simulink model "Sim_v19_PL0001_checkSignConv"  (R2015a)
settings: Solver=ode4  StartTime=0.0  StopTime=300  FixedStep=Ts  RelTol=1e-3
PreLoadFcn:
  | Ts=0.1;
PostLoadFcn:
  | Ts=0.1;
InitFcn:
  | Ts=0.1;
StartFcn:
  | Ts=0.1;
values from neighbouring files (symbols this model uses):
  ctrl_idx = strToIdx(actStr,loadNames)    [Driver_PL0001.m]
  dbc_idx = strToIdx(dbcStr,loadNames)    [Driver_PL0001.m]
  Ki_vang = Ki_vang*5    [Driver_PL0001.m]    (also in afunc.m = zeros(r,1))
  Ki_vmag = Ki_vmag*5    [Driver_PL0001.m]    (also in afunc.m = zeros(r,1))
  Kp_vang = Kp_vang*5    [Driver_PL0001.m]    (also in afunc.m = zeros(r,1))
  Kp_vmag = Kp_vmag*5    [Driver_PL0001.m]    (also in afunc.m = zeros(r,1))
  meas_idx = strToIdx(measStr,busNames)    [Driver_PL0001.m]
  ridx = ridx(~isnan(ridx))    [Driver_PL0001.m]
  Sinv = repmat(Sinv_str,1,length(ctrl_idx)/2)    [Driver_PL0001.m]
  Vang_ctrlStart = (20+80*r)*Ts    [Driver_PL0001.m]
  vang_init_actual = vang_new(4,:)    [Driver_PL0001.m]    (also in PlotLocalCtrl_May15.m = [[0:60:(minEnd-minStart)*60]',repmat(vang_new(2,:),minEnd-mi; PlotLocalCtrl_May15_2ph.m = [[0:60:(minEnd-minStart)*60]',repmat(vang_new(2,:),minEnd-mi; set_const_target.m = Vang_nom)
  Vmag_ctrlStart = (20+80*r)*Ts    [Driver_PL0001.m]
  vmag_init_actual = vmag_new(4,:)    [Driver_PL0001.m]    (also in PlotLocalCtrl_May15.m = [[0:60:(minEnd-minStart)*60]',repmat(vmag_new(2,:),minEnd-mi; PlotLocalCtrl_May15_2ph.m = [[0:60:(minEnd-minStart)*60]',repmat(vmag_new(2,:),minEnd-mi; set_const_target.m = Vmag_nom)
undefined symbols (not defined in the file or in its folder): Sbase, V1base
libraries: dspindex x9, opal_lib x2, rtlab x2, rtlab_phasor x1
settings Model: Creator=Jaimie.Swartz  LastModifiedBy=Jaimie.Swartz
settings SolverCC: AlgebraicLoopSolver=LineSearch
settings DataIOCC: SignalLoggingSaveFormat=ModelDataLogs  SignalLogging=off  DSMLogging=off  VisualizeSimOutput=off
settings OptimizationCC: ExpressionDepthLimit=2147483647
settings DebuggingCC: UnderspecifiedInitializationDetection=Classic  MergeDetectMultiDrivingBlocksExec=none  SolverPrmCheckMsg=warning  FcnCallInpInsideContextMsg=EnableAllAsWarning  StateNameClashWarn=warning
settings GRTTargetCC: CombineOutputUpdateFcns=off  GRTInterface=on

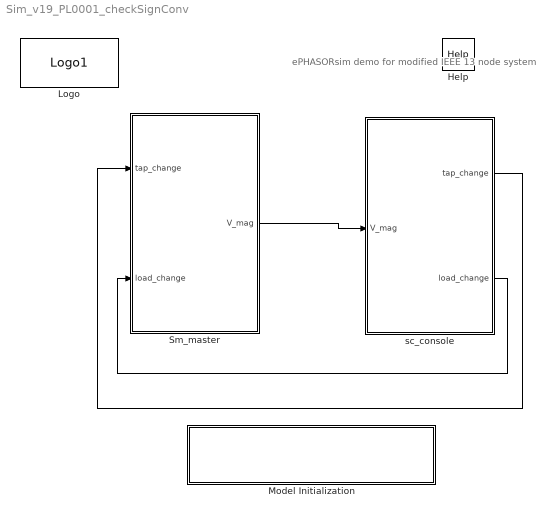
== system Sim_v19_PL0001_checkSignConv ==
  note: ePHASORsim demo for
      | modified IEEE 13 node system
  Help : opal_lib/Help  docfile=../help/ePH_IEEE13.html
  Logo : opal_lib/Logo1  vide=[]
  Model Initialization : Subsystem  mask(Model Functions){InitFcnX=Ts=0.1;, prel=on, posl=on, inif=on, strf=on}
      mask prompts: InitFcnX "Initialisation"; prel "Preload Function"; posl "PostLoad Function"; inif "InitFcn"; strf "StartFcn"
      mask init:
      | currentBlock = gcb;
      | root = bdroot(currentBlock);
      | 
      | if ~strcmp(get_param(root,'BlockDiagramType'),'library')
      |     if prel==1
      |         set_param(root, 'PreLoadFcn', InitFcnX);
      |     else
      |         set_param(root, 'PreLoadFcn', '');
      |     end
      |     if inif==1
      |         set_param(root, 'InitFcn', InitFcnX);
      |     else
      |         set_param(root, 'InitFcn', '');
      |     end
      |     if strf==1
      |         set_param(root, 'StartFcn', InitFcnX);
      |     else
      |         set_param(root, 'StartFcn', '');
      |     end
      |     if posl==1
      |         set_param(root, 'PostLoadFcn', InitFcnX);
      |     else
      |         set_param(root, 'PostLoadFcn', '');
      |     end
      | end
      | 
      | pos = get_param(currentBlock, 'Position');
      | width = pos(3) - pos(1); height = pos(4) - pos(2);
      | txt = [ upper(root) '\n' '- InitFcn. . . . . '  get_param(root, 'InitFcn') ];
      settings: CopyFcn=set_param(gcb,'LinkStatus','none')
      mask Display: text(5, height*0.5, txt, 'horizontalAlignment', 'left', 'verticalAlignment', 'middle') ;
  Sm_master : Subsystem
  sc_console : Subsystem
  wires:
  Sm_master/1(V_mag) -> sc_console/1(V_mag)
  sc_console/1(tap_change) -> Sm_master/1(tap_change)
  sc_console/2(load_change) -> Sm_master/2(load_change)

== system Sim_v19_PL0001_checkSignConv/Model Initialization ==

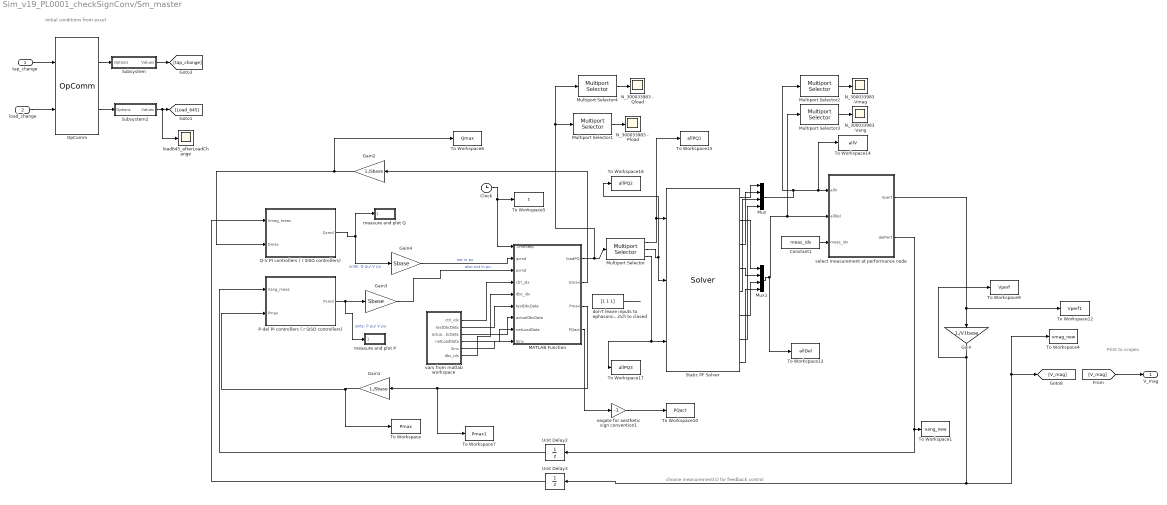
== system Sim_v19_PL0001_checkSignConv/Sm_master ==
  note: Initial conditions from excel
  note: choose measurement(s) for feedback control
  note: Print to scopes
  tap_change : Inport
  load_change : Inport  Port=2
  Clock : Clock
  Constant1 : Constant  Value=meas_idx
  Gain : Gain  Gain=1./V1base
  Gain1 : Gain  Gain=1./Sbase
  Gain2 : Gain  Gain=1./Sbase
  Gain3 : Gain  Gain=Sbase
  Gain4 : Gain  Gain=Sbase
  MATLAB Function : MATLAB Function  TreatAsAtomicUnit=on
  Multiport Selector : dspindex/Multiport Selector  rowsOrCols=Rows  idxCellArray={ [1:254], [255: 508], [509:606]}  idxErrMode=Clip Index
  Multiport Selector1 : dspindex/Multiport Selector  rowsOrCols=Rows  idxCellArray={ [1:3]}  idxErrMode=Clip Index
  Multiport Selector2 : dspindex/Multiport Selector  rowsOrCols=Rows  idxCellArray={ [577:579]}  idxErrMode=Clip Index
  Multiport Selector3 : dspindex/Multiport Selector  rowsOrCols=Rows  idxCellArray={ [577:579]}  idxErrMode=Clip Index
  Multiport Selector4 : dspindex/Multiport Selector  rowsOrCols=Rows  idxCellArray={ [304:306]}  idxErrMode=Clip Index
  Mux : Mux
  Mux1 : Mux
  N_300033983 - Pload : Scope
      settings: SaveName=ScopeData5
  N_300033983 - Qload : Scope
      settings: SaveName=ScopeData11
  N_300033983 -Vang : Scope
      settings: SaveName=ScopeData7
  N_300033983 -Vmag : Scope
      settings: SaveName=ScopeData10
  OpComm : rtlab/OpComm  nbport=2  groupe_acq=1  subsys_rate=0  st=0  Synchronization=on  Interpolation=on  Threshold=1.0  Missed_Data=off  Sim_Time=off  Samples=off  dynSigOut=off  from_console=1  warning_done=off  writeOpCommFile=off  Offset=off
  P-del PI controllers ( r SISO controllers) : Subsystem
  Q-V PI controllers ( r SISO controllers) : Subsystem
  Static PF Solver : rtlab_phasor/Solver  epname=System  extension=Excel  xls='PL0001_OPAL_working_simple.xlsx'  raw='4992b.raw'  dyr='4992b.dyr'  cyme='ieee13.sxst'  powerfactory='network.dgs'  builtin=on  cyme_pf=''  cyme_unbalanced=on  lazy_netlist=off  capidir='CAPI'  fmudir='FMU'  capiprefix=capicomp_  fmuprefix=fmucomp_  logging=off  sim_mode=Dynamic simulation only (without power-flow)  pf_max_it=100  pf_tol_v=0.00001  pf_flat_start=off  pf_smart_start=off  pf_export=on  np=1  exporty=off  dt=Ts  optim_threads=off  perflog_on=off  script_activate_postinit=off  script_postinit_name=''
  Subsystem : Subsystem
  Subsystem2 : Subsystem
  To Workspace : ToWorkspace  VariableName=Pmax  SampleTime=-1
  To Workspace1 : ToWorkspace  VariableName=vang_new  SampleTime=-1
      settings: Save2DSignal=2-D array (concatenate along first dimension)
  To Workspace10 : ToWorkspace  VariableName=PQact  SampleTime=-1
  To Workspace12 : ToWorkspace  VariableName=Vperf1  SampleTime=-1
      settings: Save2DSignal=2-D array (concatenate along first dimension)
  To Workspace13 : ToWorkspace  VariableName=allDel  SampleTime=-1
  To Workspace14 : ToWorkspace  VariableName=allV  SampleTime=-1
  To Workspace15 : ToWorkspace  VariableName=allPQ1  SampleTime=-1
      settings: Save2DSignal=2-D array (concatenate along first dimension)
  To Workspace16 : ToWorkspace  VariableName=allPQ2  SampleTime=-1
      settings: Save2DSignal=2-D array (concatenate along first dimension)
  To Workspace17 : ToWorkspace  VariableName=allPQ3  SampleTime=-1
      settings: Save2DSignal=2-D array (concatenate along first dimension)
  To Workspace4 : ToWorkspace  VariableName=vmag_new  SampleTime=-1
      settings: Save2DSignal=2-D array (concatenate along first dimension)
  To Workspace5 : ToWorkspace  VariableName=t  SampleTime=-1
      settings: Save2DSignal=2-D array (concatenate along first dimension)
  To Workspace6 : ToWorkspace  VariableName=Qmax  SampleTime=-1
  To Workspace7 : ToWorkspace  VariableName=Pmax1  SampleTime=-1
  To Workspace9 : ToWorkspace  VariableName=Vperf  SampleTime=-1
      settings: Save2DSignal=2-D array (concatenate along first dimension)
  Unit Delay2 : UnitDelay  InitialCondition=vang_init_actual  SampleTime=Ts
  Unit Delay3 : UnitDelay  InitialCondition=vmag_init_actual  SampleTime=Ts
  "don't leave inputs to ephasorsim open, takes on default val of 0 [1 1 1] sets default switch to closed" : Constant  Value=[1 1 1]
  load645_afterLoadChange : Scope
      settings: ShowLegends=on  YMin=0.94469  YMax=1.0518  SaveName=ScopeData17
  measure and plot P : Subsystem
  measure and plot Q : Subsystem
  negate for aesthetic sign convention1 : Gain  Gain=-1
  select measurement at performance node : MATLAB Function  TreatAsAtomicUnit=on
  vars from matlab workspace : Subsystem
  V_mag : Outport
  wires:
  tap_change/1 -> OpComm/1
  load_change/1 -> OpComm/2
  [V_mag] -> V_mag/1
  OpComm/1 -> Subsystem/1(Options)
  OpComm/2 -> Subsystem2/1(Options)
  Subsystem/1(Values) -> [tap_change]
  Subsystem2/1(Values) -> load645_afterLoadChange/1, [Load_645]
  Unit Delay3/1 -> Q-V PI controllers ( r SISO controllers)/1(Vmag_meas)
  vars from matlab workspace/1("ctrl_idx ") -> MATLAB Function/4(ctrl_idx)
  Constant1/1 -> select measurement at performance node/3(meas_idx)
  vars from matlab workspace/4(netLoadData) -> MATLAB Function/8(netLoadData)
  Clock/1 -> To Workspace5/1, MATLAB Function/1(TimeStep)
  vars from matlab workspace/5(Sinv) -> MATLAB Function/9(Sinv)
  Unit Delay2/1 -> P-del PI controllers ( r SISO controllers)/1(Vang_meas)
  select measurement at performance node/2(delPerf) -> Unit Delay2/1, To Workspace1/1
  MATLAB Function/2(Qmax) -> Gain2/1
  Gain4/1 -> MATLAB Function/2(qcmd)  "not in pu"
  Gain3/1 -> MATLAB Function/3(pcmd)  "also not in pu"
  Gain/1 -> To Workspace9/1, To Workspace4/1, [V_mag], Unit Delay3/1
  vars from matlab workspace/6(dbc_idx) -> MATLAB Function/5(dbc_idx)
  vars from matlab workspace/2(testDbcData) -> MATLAB Function/6(testDbcData)
  vars from matlab workspace/3(actualDbcData) -> MATLAB Function/7(actualDbcData)
  Gain1/1 -> P-del PI controllers ( r SISO controllers)/2(Pmax), To Workspace/1
  select measurement at performance node/1(Vperf) -> Gain/1, To Workspace12/1
  Gain2/1 -> Q-V PI controllers ( r SISO controllers)/2(Qmax), To Workspace6/1
  MATLAB Function/3(Pmax) -> To Workspace7/1, Gain1/1
  "don't leave inputs to ephasorsim open, takes on default val of 0 [1 1 1] sets default switch to closed"/1 -> ?
  MATLAB Function/4(PQact) -> negate for aesthetic sign convention1/1
  Q-V PI controllers ( r SISO controllers)/1(Qcmd) -> measure and plot Q/1(Qactual), Gain4/1  "units: Q pu/ V pu"
  P-del PI controllers ( r SISO controllers)/1(Pcmd) -> Gain3/1, measure and plot P/1(Pactual)  "units: P pu/ V pu"
  Mux1/1 -> To Workspace13/1, Multiport Selector3/1, select measurement at performance node/2(allDel)
  Static PF Solver/2 -> Mux1/1
  Static PF Solver/4 -> Mux1/2
  Static PF Solver/6 -> Mux1/3
  Static PF Solver/8 -> Mux1/4
  Static PF Solver/1 -> Mux/1
  Static PF Solver/3 -> Mux/2
  Static PF Solver/5 -> Mux/3
  Static PF Solver/7 -> Mux/4
  Multiport Selector/1 -> Static PF Solver/1, To Workspace15/1
  Multiport Selector/2 -> Static PF Solver/2, To Workspace16/1
  Multiport Selector/3 -> Static PF Solver/3, To Workspace17/1
  negate for aesthetic sign convention1/1 -> To Workspace10/1
  Multiport Selector1/1 -> N_300033983 - Pload/1
  Multiport Selector2/1 -> N_300033983 -Vmag/1
  Mux/1 -> To Workspace14/1, select measurement at performance node/1(allV), Multiport Selector2/1
  Multiport Selector3/1 -> N_300033983 -Vang/1
  MATLAB Function/1(loadPQ) -> Multiport Selector4/1, Multiport Selector1/1, Multiport Selector/1
  Multiport Selector4/1 -> N_300033983 - Qload/1

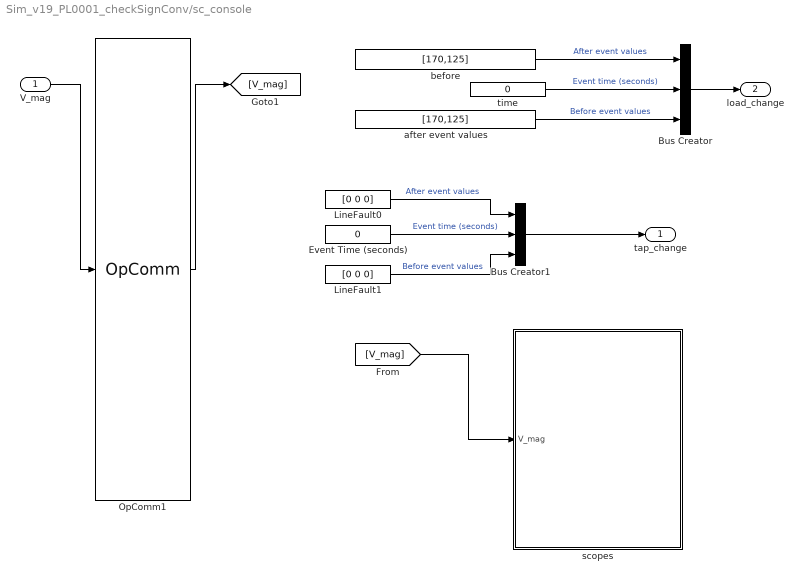
== system Sim_v19_PL0001_checkSignConv/sc_console ==
  V_mag : Inport
  Bus Creator : BusCreator  Inputs=3
  Bus Creator1 : BusCreator  Inputs=3
  Event Time (seconds) : Constant  Value=0
  LineFault0 : Constant  Value=[0 0 0]
  LineFault1 : Constant  Value=[0 0 0]
  OpComm1 : rtlab/OpComm  nbport=1  groupe_acq=1  subsys_rate=0  st=0  Synchronization=on  Interpolation=on  Threshold=1.0  Missed_Data=off  Sim_Time=off  Samples=off  dynSigOut=off  from_console=0  warning_done=off  writeOpCommFile=off  Offset=off
  after event values : Constant  Value=[170,125]
  before : Constant  Value=[170,125]
  scopes : Subsystem
  time : Constant  Value=0
  tap_change : Outport
  load_change : Outport  Port=2
  wires:
  V_mag/1 -> OpComm1/1
  OpComm1/1 -> [V_mag]
  time/1 -> Bus Creator/2  "Event time (seconds)"
  Bus Creator/1 -> load_change/1
  LineFault0/1 -> Bus Creator1/1  "After event values"
  LineFault1/1 -> Bus Creator1/3  "Before event values"
  Event Time (seconds)/1 -> Bus Creator1/2  "Event time (seconds)"
  Bus Creator1/1 -> tap_change/1
  before/1 -> Bus Creator/1  "After event values"
  after event values/1 -> Bus Creator/3  "Before event values"
  [V_mag] -> scopes/1(V_mag)

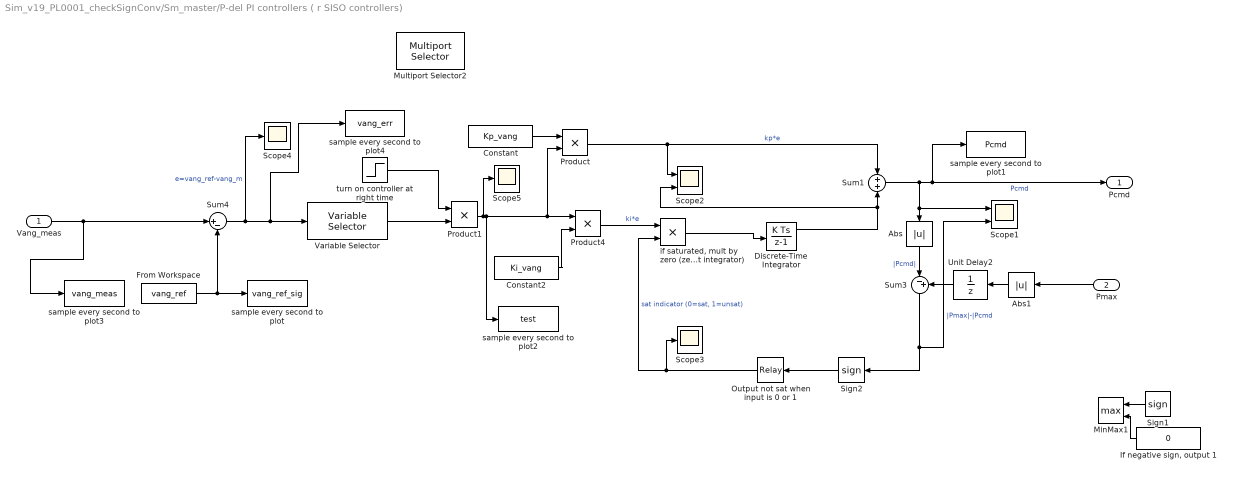
== system Sim_v19_PL0001_checkSignConv/Sm_master/P-del PI controllers ( r SISO controllers) ==
  Vang_meas : Inport
  Pmax : Inport  Port=2
  Abs : Abs
  Abs1 : Abs
  Constant : Constant  Value=Kp_vang
  Constant2 : Constant  Value=Ki_vang
  Discrete-Time Integrator : DiscreteIntegrator  gainval=1  InitialConditionSetting=State (most efficient)  SampleTime=Ts  ShowSaturationPort=on
  From Workspace : FromWorkspace  VariableName=vang_ref  SampleTime=0
  "If negative sign, output 1" : Constant  Value=0
  MinMax1 : MinMax  Function=max  Inputs=2
  Multiport Selector2 : dspindex/Multiport Selector  rowsOrCols=Columns  idxCellArray={ridx}  idxErrMode=Clip Index
  "Output not sat when input is 0 or 1 " : Relay  OnSwitchValue=-0.5  OffSwitchValue=-0.5
  Product : Product
  Product1 : Product
  Product4 : Product
  Scope1 : Scope  NumInputPorts=2
      settings: ShowLegends=on  YMin=-46.25~-5  YMax=6.25~5  SaveName=ScopeData8
  Scope2 : Scope  NumInputPorts=2
      settings: YMin=-23.625~-5  YMax=2.625~5  SaveName=ScopeData2
  Scope3 : Scope
      settings: ShowLegends=on  YMin=-0.125  YMax=1.125  SaveName=ScopeData9
  Scope4 : Scope
      settings: YMin=-0.125  YMax=1.125
  Scope5 : Scope
      settings: ShowLegends=on  YMin=-0.125  YMax=1.125  SaveName=ScopeData3  ScrollMode=on
  Sign1 : Signum
  Sign2 : Signum
  Sum1 : Sum  Inputs=+|+
  Sum3 : Sum  Inputs=|-+
  Sum4 : Sum  Inputs=|+-
  Unit Delay2 : UnitDelay  InitialCondition=Sinv  SampleTime=Ts
  Variable Selector : dspindex/Variable Selector  NumInputs=1  rowsOrCols=Columns  IdxMode=Fixed  Elements=[ridx]  ZerOneIdxMode=One-based  errmode=Clip Index  FillMode=on  FillValues=0
  "if saturated, mult by zero (zero out integrator)" : Product
  sample every second to plot : ToWorkspace  VariableName=vang_ref_sig  SampleTime=-1
  sample every second to plot1 : ToWorkspace  VariableName=Pcmd  SampleTime=-1
  sample every second to plot2 : ToWorkspace  VariableName=test  SampleTime=-1
  sample every second to plot3 : ToWorkspace  VariableName=vang_meas  SampleTime=-1
  sample every second to plot4 : ToWorkspace  VariableName=vang_err  SampleTime=-1
  turn on controller at right time : Step  Time=Vang_ctrlStart  SampleTime=0
  Pcmd : Outport
  wires:
  Sum4/1 -> Variable Selector/1, sample every second to plot4/1, Scope4/1  "e=vang_ref-vang_m"
  Constant/1 -> Product/1
  turn on controller at right time/1 -> Product1/1
  Product1/1 -> Product/2, Product4/1, sample every second to plot2/1, Scope5/1
  Constant2/1 -> Product4/2
  Product/1 -> Scope2/1, Sum1/1  "kp*e"
  Sum1/1 -> Abs/1, Scope1/1, sample every second to plot1/1, Pcmd/1  "Pcmd"
  Sum3/1 -> Sign2/1, Scope1/2  "|Pmax|-|Pcmd"
  "if saturated, mult by zero (zero out integrator)"/1 -> Discrete-Time Integrator/1
  Product4/1 -> "if saturated, mult by zero (zero out integrator)"/1  "ki*e"
  Pmax/1 -> Abs1/1
  Abs/1 -> Sum3/1  "|Pcmd|"
  "Output not sat when input is 0 or 1 "/1 -> Scope3/1, "if saturated, mult by zero (zero out integrator)"/2  "sat indicator (0=sat, 1=unsat)"
  Discrete-Time Integrator/1 -> Scope2/2, Sum1/2
  Unit Delay2/1 -> Sum3/2
  Abs1/1 -> Unit Delay2/1
  Vang_meas/1 -> Sum4/1, sample every second to plot3/1
  From Workspace/1 -> Sum4/2, sample every second to plot/1
  Variable Selector/1 -> Product1/2
  Sign1/1 -> MinMax1/1
  "If negative sign, output 1"/1 -> MinMax1/2
  Sign2/1 -> "Output not sat when input is 0 or 1 "/1

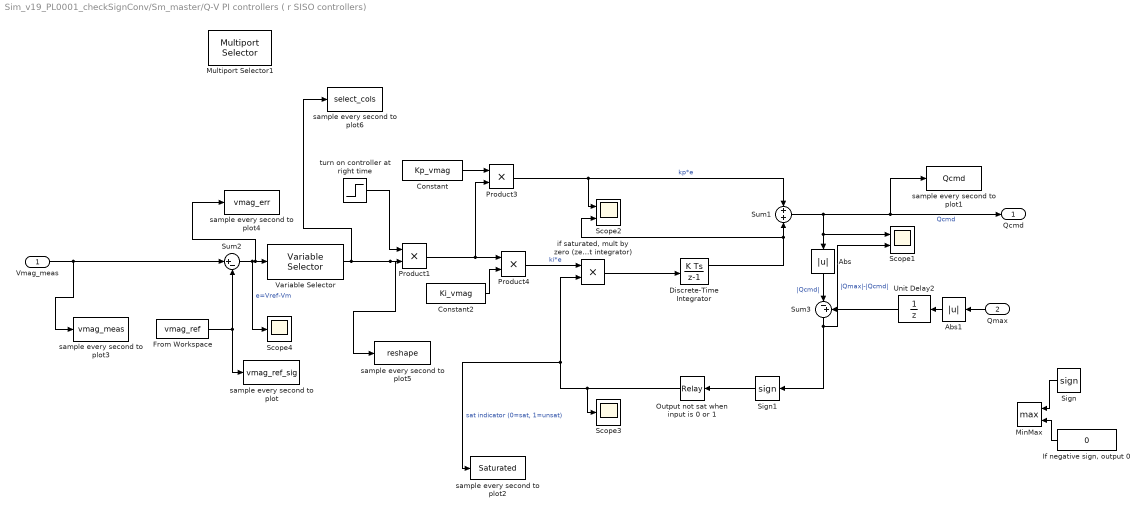
== system Sim_v19_PL0001_checkSignConv/Sm_master/Q-V PI controllers ( r SISO controllers) ==
  Vmag_meas : Inport
  Qmax : Inport  Port=2
  Abs : Abs
  Abs1 : Abs
  Constant : Constant  Value=Kp_vmag
  Constant2 : Constant  Value=Ki_vmag
  Discrete-Time Integrator : DiscreteIntegrator  gainval=1  InitialConditionSetting=State (most efficient)  SampleTime=Ts  ShowSaturationPort=on
  From Workspace : FromWorkspace  VariableName=vmag_ref  SampleTime=0
  "If negative sign, output 0" : Constant  Value=0
  MinMax : MinMax  Function=max  Inputs=2
  Multiport Selector1 : dspindex/Multiport Selector  rowsOrCols=Columns  idxCellArray={ridx}  idxErrMode=Clip Index
  Output not sat when input is 0 or 1 : Relay  OnSwitchValue=-0.5  OffSwitchValue=-0.5
  Product1 : Product
  Product3 : Product
  Product4 : Product
  Scope1 : Scope  NumInputPorts=2
      settings: ShowLegends=on  YMin=-46.25~-5  YMax=6.25~5  SaveName=ScopeData8
  Scope2 : Scope  NumInputPorts=2
      settings: ShowLegends=on  YMin=-23.625~-5  YMax=2.625~5  SaveName=ScopeData2
  Scope3 : Scope
      settings: ShowLegends=on  YMin=-0.125  YMax=1.125  SaveName=ScopeData9
  Scope4 : Scope
      settings: ShowLegends=on  YMin=-0.125  YMax=1.125  SaveName=ScopeData4
  Sign : Signum
  Sign1 : Signum
  Sum1 : Sum  Inputs=+|+
  Sum2 : Sum  Inputs=|+-
  Sum3 : Sum  Inputs=|-+
  Unit Delay2 : UnitDelay  InitialCondition=Sinv  SampleTime=Ts
  Variable Selector : dspindex/Variable Selector  NumInputs=1  rowsOrCols=Columns  IdxMode=Fixed  Elements=[ridx]  ZerOneIdxMode=One-based  errmode=Clip Index  FillMode=on  FillValues=0
  "if saturated, mult by zero (zero out integrator)" : Product
  sample every second to plot : ToWorkspace  VariableName=vmag_ref_sig  SampleTime=-1
  sample every second to plot1 : ToWorkspace  VariableName=Qcmd  SampleTime=-1
  sample every second to plot2 : ToWorkspace  VariableName=Saturated  SampleTime=-1
  sample every second to plot3 : ToWorkspace  VariableName=vmag_meas  SampleTime=-1
  sample every second to plot4 : ToWorkspace  VariableName=vmag_err  SampleTime=-1
  sample every second to plot5 : ToWorkspace  VariableName=reshape  SampleTime=-1
  sample every second to plot6 : ToWorkspace  VariableName=select_cols  SampleTime=-1
  turn on controller at right time : Step  Time=Vmag_ctrlStart  SampleTime=0
  Qcmd : Outport
  wires:
  Sum2/1 -> Variable Selector/1, sample every second to plot4/1, Scope4/1  "e=Vref-Vm"
  Constant/1 -> Product3/1
  turn on controller at right time/1 -> Product1/1
  Product1/1 -> Product4/1, Product3/2
  Constant2/1 -> Product4/2
  Product3/1 -> Scope2/1, Sum1/1  "kp*e"
  Sum1/1 -> Abs/1, Scope1/1, sample every second to plot1/1, Qcmd/1  "Qcmd"
  Sum3/1 -> Sign1/1, Scope1/2  "|Qmax|-|Qcmd|"
  "if saturated, mult by zero (zero out integrator)"/1 -> Discrete-Time Integrator/1
  Product4/1 -> "if saturated, mult by zero (zero out integrator)"/1  "ki*e"
  Qmax/1 -> Abs1/1
  Abs/1 -> Sum3/1  "|Qcmd|"
  Output not sat when input is 0 or 1/1 -> Scope3/1, "if saturated, mult by zero (zero out integrator)"/2, sample every second to plot2/1  "sat indicator (0=sat, 1=unsat)"
  Discrete-Time Integrator/1 -> Scope2/2, Sum1/2
  Unit Delay2/1 -> Sum3/2
  Abs1/1 -> Unit Delay2/1
  Vmag_meas/1 -> Sum2/1, sample every second to plot3/1
  From Workspace/1 -> Sum2/2, sample every second to plot/1
  Variable Selector/1 -> sample every second to plot6/1, sample every second to plot5/1, Product1/2
  Sign/1 -> MinMax/1
  "If negative sign, output 0"/1 -> MinMax/2
  Sign1/1 -> Output not sat when input is 0 or 1/1

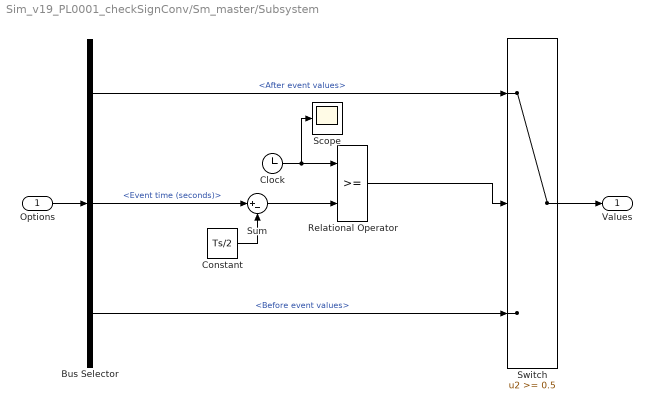
== system Sim_v19_PL0001_checkSignConv/Sm_master/Subsystem ==
  Options : Inport
  Bus Selector : BusSelector  OutputSignals=After event values,Event time (seconds),Before event values
  Clock : Clock
  Constant : Constant  Value=Ts/2
  Relational Operator : RelationalOperator  OutDataTypeStr=boolean
  Scope : Scope
  Sum : Sum  Inputs=|+-
  Switch : Switch  Threshold=0.5
  Values : Outport
  wires:
  Clock/1 -> Scope/1, Relational Operator/1
  Constant/1 -> Sum/2
  Sum/1 -> Relational Operator/2
  Bus Selector/2 -> Sum/1  "<Event time (seconds)>"
  Relational Operator/1 -> Switch/2
  Bus Selector/3 -> Switch/3  "<Before event values>"
  Bus Selector/1 -> Switch/1  "<After event values>"
  Switch/1 -> Values/1
  Options/1 -> Bus Selector/1

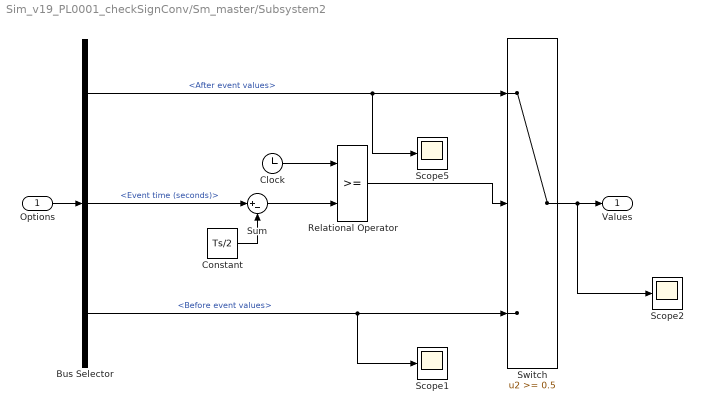
== system Sim_v19_PL0001_checkSignConv/Sm_master/Subsystem2 ==
  Options : Inport
  Bus Selector : BusSelector  OutputSignals=After event values,Event time (seconds),Before event values
  Clock : Clock
  Constant : Constant  Value=Ts/2
  Relational Operator : RelationalOperator  OutDataTypeStr=boolean
  Scope1 : Scope
      settings: SaveName=ScopeData14
  Scope2 : Scope
      settings: SaveName=ScopeData15
  Scope5 : Scope
      settings: SaveName=ScopeData13
  Sum : Sum  Inputs=|+-
  Switch : Switch  Threshold=0.5
  Values : Outport
  wires:
  Clock/1 -> Relational Operator/1
  Constant/1 -> Sum/2
  Sum/1 -> Relational Operator/2
  Bus Selector/2 -> Sum/1  "<Event time (seconds)>"
  Relational Operator/1 -> Switch/2
  Bus Selector/3 -> Switch/3, Scope1/1  "<Before event values>"
  Bus Selector/1 -> Switch/1, Scope5/1  "<After event values>"
  Switch/1 -> Values/1, Scope2/1
  Options/1 -> Bus Selector/1

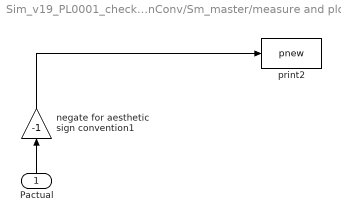
== system Sim_v19_PL0001_checkSignConv/Sm_master/measure and plot P ==
  Pactual : Inport
  negate for aesthetic sign convention1 : Gain  Gain=-1
  print2 : ToWorkspace  VariableName=pnew  SampleTime=-1
      settings: Save2DSignal=2-D array (concatenate along first dimension)
  wires:
  Pactual/1 -> negate for aesthetic sign convention1/1
  negate for aesthetic sign convention1/1 -> print2/1

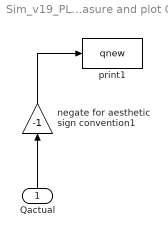
== system Sim_v19_PL0001_checkSignConv/Sm_master/measure and plot Q ==
  Qactual : Inport
  negate for aesthetic sign convention1 : Gain  Gain=-1
  print1 : ToWorkspace  VariableName=qnew  SampleTime=-1
      settings: Save2DSignal=2-D array (concatenate along first dimension)
  wires:
  Qactual/1 -> negate for aesthetic sign convention1/1
  negate for aesthetic sign convention1/1 -> print1/1

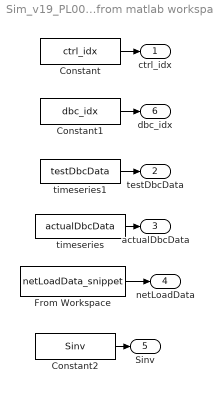
== system Sim_v19_PL0001_checkSignConv/Sm_master/vars from matlab workspace ==
  Constant : Constant  Value=ctrl_idx
  Constant1 : Constant  Value=dbc_idx
  Constant2 : Constant  Value=Sinv
  From Workspace : FromWorkspace  VariableName=netLoadData_snippet  OutDataTypeStr=double  OutputAfterFinalValue=Holding final value
  timeseries : FromWorkspace  VariableName=actualDbcData  SampleTime=0
  timeseries1 : FromWorkspace  VariableName=testDbcData  OutDataTypeStr=double  SampleTime=0
  "ctrl_idx " : Outport
  testDbcData : Outport  Port=2
  actualDbcData : Outport  Port=3
  netLoadData : Outport  Port=4
  Sinv : Outport  Port=5
  dbc_idx : Outport  Port=6
  wires:
  Constant/1 -> "ctrl_idx "/1
  Constant1/1 -> dbc_idx/1
  From Workspace/1 -> netLoadData/1
  timeseries1/1 -> testDbcData/1
  timeseries/1 -> actualDbcData/1
  Constant2/1 -> Sinv/1

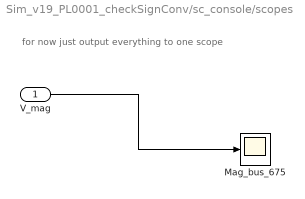
== system Sim_v19_PL0001_checkSignConv/sc_console/scopes ==
  note: for now just output everything to one scope
  V_mag : Inport
  Mag_bus_675 : Scope
      settings: YMin=0.92  YMax=1.07  SaveName=ScopeData6
  wires:
  V_mag/1 -> Mag_bus_675/1

== matlab function Sim_v19_PL0001_checkSignConv/Sm_master/select measurement at performance node ==
  data: Vperf output; allV input; allDel input; delPerf output; meas_idx input
function [Vperf,delPerf]=selectMeas(allV,allDel,meas_idx)
% use measStr,nodeNames from workspace
    Vperf=allV(meas_idx);
    delPerf=allDel(meas_idx);
end

== matlab function Sim_v19_PL0001_checkSignConv/Sm_master/MATLAB Function ==
  data: TimeStep input; qcmd input; pcmd input; loadPQ output double size=606; Qmax output; ctrl_idx input; dbc_idx input; testDbcData input; actualDbcData input; netLoadData input double size=606; Sinv input; Pmax output; PQact output
function [loadPQ, Qmax ,Pmax, PQact]  = updatePows(TimeStep, qcmd,pcmd,ctrl_idx,dbc_idx,testDbcData,actualDbcData,netLoadData,Sinv)
% netLoadData, dbcData, and k are timeseries, fed once by one for each timestep
% ctrl_idx and dbc_idx are constant
    % inputs: 
        % k is current timestep
        % 3x1 vectors of unadjusted actuation, as if have 1 actuator and it's located at the perf node 
    % inputs: rx1 vectors of powers at all nodes 
        % r is number of phases across all nodes, i.e. the dim of the pin
        % vector input to RTlab solve
%      TimeStep  % in seconds

   %% actuation signal sent from controller to devices
   %% Devices actuate here:
    % Device enforces basic inv limit by moving operating point to closest
    % point on the inv circle
    % Keith's attempt 
%     pact=zeros(1,3); qact=zeros(1,3); % initialize, TEMP, assume single actuator is on 3 phases
%     Pmax=zeros(1,3); Qmax=zeros(1,3);
%     for i=1:3 % across phases, TEMP, assuming the single actuator is on 3 phases
%         if pcmd(i)^2+qcmd(i)^2>Sinv(i)^2
%             Pmax(i)=pcmd(i)*Sinv(i)/(sqrt(pcmd(i)^2+qcmd(i)^2));
%             Qmax(i)=qcmd(i)*Sinv(i)/(sqrt(pcmd(i)^2+qcmd(i)^2));        
%             if pcmd(i) > Sinv(i)
%                 Pmax(i) = Sinv(i);
%                 Qmax(i) = 0;
%             elseif pcmd(i) < -Sinv(i)
%                 Pmax(i) = -Sinv(i); %sign?
%                 Qmax(i) = 0;
%             else
%                 Pmax(i) = pcmd(i);
%                 Qmax(i) = sqrt((Sinv(i)^2 - Pmax(i)^2)); %sign?
%             end            
%             pact(i)=Pmax(i);
%             qact(i)=Qmax(i);
%         else
%             pact(i)=pcmd(i);
%             qact(i)=qcmd(i);
%             Pmax(i) = Sinv(i);
%             Qmax(i) = Sinv(i);
%         end
%     end
% cmd=[pcmd qcmd] % print for debugging
    r = length(ctrl_idx)/2;
    %Jaimie 
    
    pact=zeros(1,r); qact=zeros(1,r); % initialize, TEMP, assume single actuator is on 3 phases
    Pmax=zeros(1,r); Qmax=zeros(1,r);
    for i=1:r % across phases, TEMP, assuming the single actuator is on 3 phases
        Pmax(i)=pcmd(i)*Sinv(i)/(sqrt(pcmd(i)^2+qcmd(i)^2));
        Qmax(i)=qcmd(i)*Sinv(i)/(sqrt(pcmd(i)^2+qcmd(i)^2)); 
        Pmax(isnan(Pmax))= 0; 
        Qmax(isnan(Qmax))= 0; 
        if pcmd(i)^2+qcmd(i)^2>Sinv(i)^2
            pact(i)= Pmax(i);
            qact(i)= Qmax(i);
        else
            pact(i)=pcmd(i);
            qact(i)=qcmd(i);
        end
    end
  
% %2.1 Topology change 
%      TopologyChangeStart=150; TopologyChangeEnd=200; %TEMP, choose this each time 
%      
%      if TopologyChangeStart <= TimeStep & TimeStep < TopologyChangeEnd  % TopologyChangeStart <=  %modify the netLoadData matrix to show the disturbance
%          switchValues = [0 0 0]; %switch opens at beginning of disturbance 
%      else
%          switchValues = [1 1 1];
%      end
     
    
%%
  
%     PQact=[pact(1) qact(1)]'; %TEMP, change for different actuator length    
    % you can print this for debugging
%     pact 
%     qact
    actpq = [pact.' qact.']; % P in first col, Q in second
    PQact = reshape(actpq,[1,length(ctrl_idx)]).'; % make col vec with Ps grouped then Qs grouped
    a=reshape(testDbcData,[2,length(ctrl_idx)/2]);
    testDbcData=reshape(a',[length(ctrl_idx),1]); % make col vec with Ps grouped then Qs grouped
    a=reshape(actualDbcData,[2,length(dbc_idx)/2]);
    actualDbcData=reshape(a',[length(dbc_idx),1]); % make col vec with Ps grouped then Qs grouped
    


    % Note: loadPQ expects P to be grouped together, then Qs
    loadPQ=zeros(size(netLoadData));
    %loadPQ = zeros(908);%TEMP     
    %disp(length(loadPQ));% just to check length
    %coder.varsize('loadPQ',[908 1]);
    %coder.varsize('netLoadData',[908 1]);
        
     
    loadPQ=netLoadData; % P&Q, ordered according to loadNames
%    if (TimeStep<5 && TimeStep>3) % in seconds
%         loadPQ(ctrl_idx)+PQact+testDbcData
%     end
    loadPQ(ctrl_idx)=loadPQ(ctrl_idx)+PQact+testDbcData;
    loadPQ(dbc_idx)=loadPQ(dbc_idx)+actualDbcData;
    
    % Note: it's ok for these values to be neg because it's NET load
end
